simulink library "SendToGES"  (R2016b)
settings: Solver=VariableStepAuto  StartTime=0.0  StopTime=10.0  RelTol=1e-3
settings Model: Creator=march  LastModifiedBy=march

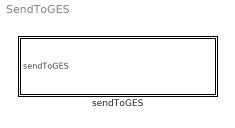
== system SendToGES ==
  sendToGES : Subsystem

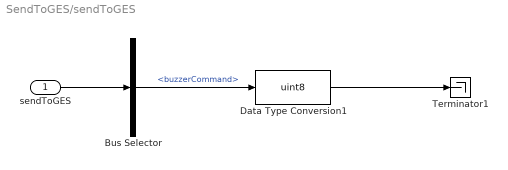
== system SendToGES/sendToGES ==
  sendToGES : Inport  OutDataTypeStr=Bus: EtherCATSendToPDB  BusOutputAsStruct=on
  Bus Selector : BusSelector  OutputSignals=buzzerCommand
  Data Type Conversion1 : DataTypeConversion  OutDataTypeStr=uint8
  Terminator1 : Terminator
  wires:
  sendToGES/1 -> Bus Selector/1
  Bus Selector/1 -> Data Type Conversion1/1  "<buzzerCommand>"
  Data Type Conversion1/1 -> Terminator1/1
